simulink model "Motor_control"  (R2017b)
settings: Solver=FixedStepDiscrete  StartTime=0.0  StopTime=50  FixedStep=0.1  RelTol=1e-3
values from neighbouring files (symbols this model uses):
  gi = Simulink.Parameter    [khoi_tao_thong_so.m]
  gp = Simulink.Parameter    [khoi_tao_thong_so.m]
  ki = Simulink.Parameter    [khoi_tao_thong_so.m]
  kp = Simulink.Parameter    [khoi_tao_thong_so.m]
libraries: simulink x1
settings Model: Creator=DELL  LastModifiedBy=DELL
settings OptimizationCC: DefaultParameterBehavior=Inlined  UseDivisionForNetSlopeComputation=on  UseFloatMulNetSlope=on  InlineInvariantSignals=on  PassReuseOutputArgsAs=Individual arguments  ZeroExternalMemoryAtStartup=off  ZeroInternalMemoryAtStartup=off  NoFixptDivByZeroProtection=on  EfficientFloat2IntCast=on  LifeSpan=1
settings DebuggingCC: ParameterTunabilityLossMsg=error
settings HardwareCC: ProdLongLongMode=on
settings SFSimCC: MATLABDynamicMemAlloc=off
settings RTWCC: SystemTargetFile=ert.tlc  GenCodeOnly=on  TemplateMakefile=ert_default_tmf  GenerateReport=on  IncludeHyperlinkInReport=on  LaunchReport=on  GenerateTraceInfo=on  GenerateTraceReport=on  GenerateTraceReportSl=on  GenerateTraceReportSf=on  GenerateTraceReportEml=on  GenerateCodeMetricsReport=on
settings CodeAppCC: ForceParamTrailComments=on  IgnoreCustomStorageClasses=off  OperatorAnnotations=on  SimulinkDataObjDesc=on  SFDataObjDesc=on  CustomSymbolStrGlobalVar=rt$N$M  CustomSymbolStrType=$N$M  CustomSymbolStrFcn=$N$M$F  CustomSymbolStrMacro=$N$M  InsertBlockDesc=on
settings ERTTargetCC: TargetLangStandard=C99 (ISO)  GenerateSampleERTMain=on  IncludeMdlTerminateFcn=off  CombineSignalStateStructs=on  SuppressErrorStatus=on  SupportAbsoluteTime=off  SupportComplex=off  InlinedParameterPlacement=NonHierarchical  ERTCustomFileTemplate=example_file_process.tlc  ERTFilePackagingFormat=CompactWithDataFile

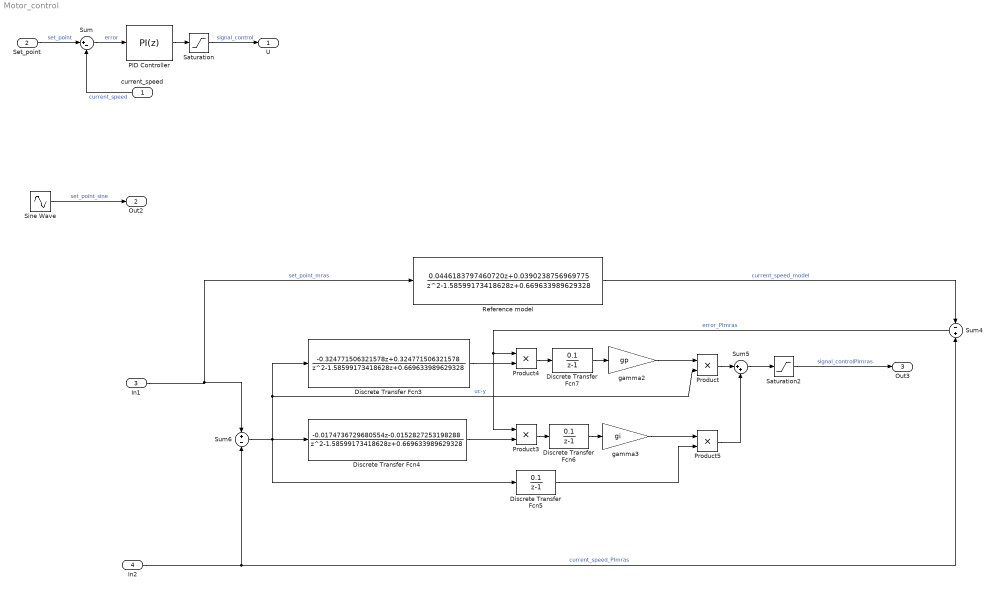
== system Motor_control ==
  current_speed : Inport
  "Set_point " : Inport  Port=2
  In1 : Inport  Port=3
  In2 : Inport  Port=4
  Discrete Transfer Fcn3 : DiscreteTransferFcn  Numerator=[0 -0.324771506321578 0.324771506321578]  Denominator=[1 -1.58599173418628 0.669633989629328]
  Discrete Transfer Fcn4 : DiscreteTransferFcn  Numerator=[0 -0.0174736729680554 -0.0152827253198288]  Denominator=[1 -1.58599173418628 0.669633989629328]
  Discrete Transfer Fcn5 : DiscreteTransferFcn  Numerator=[0.1]  Denominator=[1 -1]
  Discrete Transfer Fcn6 : DiscreteTransferFcn  Numerator=[0.1]  Denominator=[1 -1]
  Discrete Transfer Fcn7 : DiscreteTransferFcn  Numerator=[0.1]  Denominator=[1 -1]
  PID Controller : simulink/Continuous/PID Controller  Controller=PI  TimeDomain=Discrete-time  SampleTime=-1  IntegratorMethod=Forward Euler  FilterMethod=Forward Euler  Form=Parallel  UseFilter=off  ControllerParametersSource=internal  P=kp  I=ki  D=0  N=100  InitialConditionSource=internal  InitialConditionForIntegrator=0  InitialConditionForFilter=0  ExternalReset=none  LimitOutput=off  UpperSaturationLimit=inf  LowerSaturationLimit=-inf  LinearizeAsGain=on  AntiWindupMode=none  Kb=1  TrackingMode=off  Kt=1  PParamMin=[]  PParamMax=[]  IParamMin=[]  IParamMax=[]  DParamMin=[]  DParamMax=[]  NParamMin=[]  NParamMax=[]  KbParamMin=[]  KbParamMax=[]  KtParamMin=[]  KtParamMax=[]  POutMin=[]  POutMax=[]  IOutMin=[]  IOutMax=[]  DOutMin=[]  DOutMax=[]  NOutMin=[]  NOutMax=[]  KbOutMin=[]  KbOutMax=[]  KtOutMin=[]  KtOutMax=[]  IntegratorOutMin=[]  IntegratorOutMax=[]  FilterOutMin=[]  FilterOutMax=[]  SumOutMin=[]  SumOutMax=[]  SumI1OutMin=[]  SumI1OutMax=[]  SumI2OutMin=[]  SumI2OutMax=[]  SumI3OutMin=[]  SumI3OutMax=[]  SumDOutMin=[]  SumDOutMax=[]  SaturationOutMin=[]  SaturationOutMax=[]  IntegratorContinuousStateAttributes=''  IntegratorStateMustResolveToSignalObject=off  IntegratorRTWStateStorageClass=Auto  FilterContinuousStateAttributes=''  FilterStateMustResolveToSignalObject=off  FilterRTWStateStorageClass=Auto  DifferentiatorICPrevScaledInput=0  DifferentiatorOutMin=[]  DifferentiatorOutMax=[]  InitialConditionSetting=State (most efficient)  FilterDiffOutCoefMin=[]  FilterDiffOutCoefMax=[]  SumDenOutMin=[]  SumDenOutMax=[]  SumNumOutMin=[]  SumNumOutMax=[]  ReciprocalOutMin=[]  ReciprocalOutMax=[]  DivideOutMin=[]  DivideOutMax=[]  TunerSelectOption=Transfer Function Based (PID Tuner App)
  Product{,3..5} (4 alike) : Product
  Reference model : DiscreteTransferFcn  Numerator=[0 0.0446183797460720 0.0390238756969775]  Denominator=[1,-1.58599173418628,0.669633989629328]
  Saturation : Saturate  UpperLimit=100  LowerLimit=0
  Saturation2 : Saturate  UpperLimit=100  LowerLimit=0
  Sine Wave : Sin  SineType=Sample based  Amplitude=100  Bias=150  Samples=9999  SampleTime=0.1
  Sum : Sum  Inputs=|+-
  Sum4 : Sum  Inputs=-|+
  Sum5 : Sum  Inputs=|++
  Sum6 : Sum  Inputs=+|-
  gamma2 : Gain  Gain=gp
  gamma3 : Gain  Gain=gi
  U : Outport
  Out2 : Outport  Port=2
  Out3 : Outport  Port=3
  wires:
  current_speed/1 -> Sum/2  "current_speed"
  Sum/1 -> PID Controller/1  "error"
  "Set_point "/1 -> Sum/1  "set_point"
  Saturation/1 -> U/1  "signal_control"
  PID Controller/1 -> Saturation/1
  Sine Wave/1 -> Out2/1  "set_point_sine"
  Sum4/1 -> Product3/1, Product4/1  "error_PImras"
  Discrete Transfer Fcn6/1 -> gamma3/1
  gamma3/1 -> Product5/1
  Discrete Transfer Fcn4/1 -> Product3/2
  gamma2/1 -> Product/1
  Discrete Transfer Fcn7/1 -> gamma2/1
  Product3/1 -> Discrete Transfer Fcn6/1
  Discrete Transfer Fcn3/1 -> Product4/2
  Product/1 -> Sum5/1
  Reference model/1 -> Sum4/1  "current_speed_model"
  Product5/1 -> Sum5/2
  Discrete Transfer Fcn5/1 -> Product5/2
  Sum5/1 -> Saturation2/1
  Product4/1 -> Discrete Transfer Fcn7/1
  Sum6/1 -> Discrete Transfer Fcn5/1, Discrete Transfer Fcn3/1, Product/2, Discrete Transfer Fcn4/1  "uc-y"
  In1/1 -> Sum6/1, Reference model/1  "set_point_mras"
  In2/1 -> Sum6/2, Sum4/2  "current_speed_PImras"
  Saturation2/1 -> Out3/1  "signal_controlPImras"
